simulink model "observerModel_MS"  (R2023b)
settings: Solver=ode15s  StartTime=0.0  StopTime=duration  MaxStep=0.02  RelTol=0.02  AbsTol=0.02  EnableMultiTasking=on
values from neighbouring files (symbols this model uses):
  beta1 = s(8)    [Observer_Optimize.m]
  beta2 = s(7)    [Observer_Optimize.m]
  delta_t = time(2) - time (1)    [Observer_Optimize.m]
  df = 1    [Observer_Optimize.m]
  f_oto = 2    [Observer_Optimize.m]
  f_scc = 2    [Observer_Optimize.m]
  f_visO = 0.2    [Observer_Optimize.m]
  f_visV = 2    [Observer_Optimize.m]
  f_visX = 2    [Observer_Optimize.m]
  GG0 = [0 0 -hypo]'    [Observer_Optimize.m]
  kaa = -2*[1 1 1]'    [Observer_Optimize.m]
  Kea = s(1)^(1/2)*[1 1 1]    [Observer_Optimize.m]
  Kef = s(3)^(1/2)*[1 1 1]    [Observer_Optimize.m]
  Kew = s(2)^(1/2)*[1 1 1]    [Observer_Optimize.m]
  Kfast = s(4)    [Observer_Optimize.m]
  kfg = 1*[1 1 1]'    [Observer_Optimize.m]
  kfw = 1*[1 1 1]'    [Observer_Optimize.m]
  kgvg = 5*[1 1 1]'    [Observer_Optimize.m]
  kwg = 1*[1 1 1]'    [Observer_Optimize.m]
  kwvw = 10*[1 1 1]'    [Observer_Optimize.m]
  kww = 3*[1 1 1]'    [Observer_Optimize.m]
  kxdotva = 0.75*[1 1 1]'    [Observer_Optimize.m]
  kxvv = 0.1*[1 1 1]'    [Observer_Optimize.m]
  ms_exp = s(6)    [Observer_Optimize.m]
  oto_a = 60*[1 1 1]'    [Observer_Optimize.m]
  oto_Ka = 1.3*[1 1 1]'    [Observer_Optimize.m]
  Q0 = [cos(E_angle/2) E(1)*sin(E_angle/2) E(2)*sin(E_angle/2) E(3)*sin(E_angle/2)]'    [Observer_Optimize.m]
  tau_a = tau_a_value*[1 1 1]'    [Observer_Optimize.m]
  tau_scc = tau_scc_value*[1 1 1]'    [Observer_Optimize.m]
  x_leak = 0.6    [Observer_Optimize.m]
  y_leak = 0.6    [Observer_Optimize.m]
  z_leak = 10    [Observer_Optimize.m]
(part 1 of 3)
settings Model: Creator=Newman  LastModifiedBy=aaronallred
settings SolverCC: AutoScaleAbsTol=off  AlgebraicLoopSolver=TrustRegion
settings DataIOCC: SaveFormat=Array  SignalLoggingSaveFormat=ModelDataLogs  SaveOutput=off  SaveTime=off  ReturnWorkspaceOutputs=off
settings OptimizationCC: ExpressionDepthLimit=2147483647  InitFltsAndDblsToZero=on  LifeSpan=inf
settings DebuggingCC: SaveWithParameterizedLinksMsg=none  UnderspecifiedInitializationDetection=Classic  MergeDetectMultiDrivingBlocksExec=none  SolverPrmCheckMsg=warning  FcnCallInpInsideContextMsg=warning  UnconnectedInputMsg=warning  UnconnectedOutputMsg=warning  UnconnectedLineMsg=warning  StateNameClashWarn=warning  SFUnexpectedBacktrackingDiag=warning  SFNoUnconditionalDefaultTransitionDiag=warning  SFExecutionAtInitializationDiag=none  ArithmeticOperatorsInVariantConditions=warning
settings HardwareCC: ProdBitPerPointer=32  ProdBitPerSizeT=32  ProdBitPerPtrDiffT=32  ProdLargestAtomicFloat=None  ProdIntDivRoundTo=Undefined  ProdEndianess=Unspecified  ProdWordSize=32  ProdHWDeviceType=32-bit Generic
settings ModelReferenceCC: EnableRefExpFcnMdlSchedulingChecks=on  PropagateSignalLabelsOutOfModel=off
settings SFSimCC: SimUseLocalCustomCode=off  CustomCodeUndefinedFunction=UseInterfaceOnly
settings RTWCC: RTWUseLocalCustomCode=off  DLArmComputeVersion=19.05
settings CodeAppCC: StateflowObjectComments=on
settings GRTTargetCC: TargetFcnLib=ansi_tfl_tmw.mat  TargetLangStandard=C89/C90 (ANSI)  CombineOutputUpdateFcns=off  GRTInterface=on
settings ConfigComp: CovMetricSettings=dw  CovSaveCumulativeToWorkspaceVar=on  CovSaveSingleToWorkspaceVar=on  CovExternalEMLEnable=off

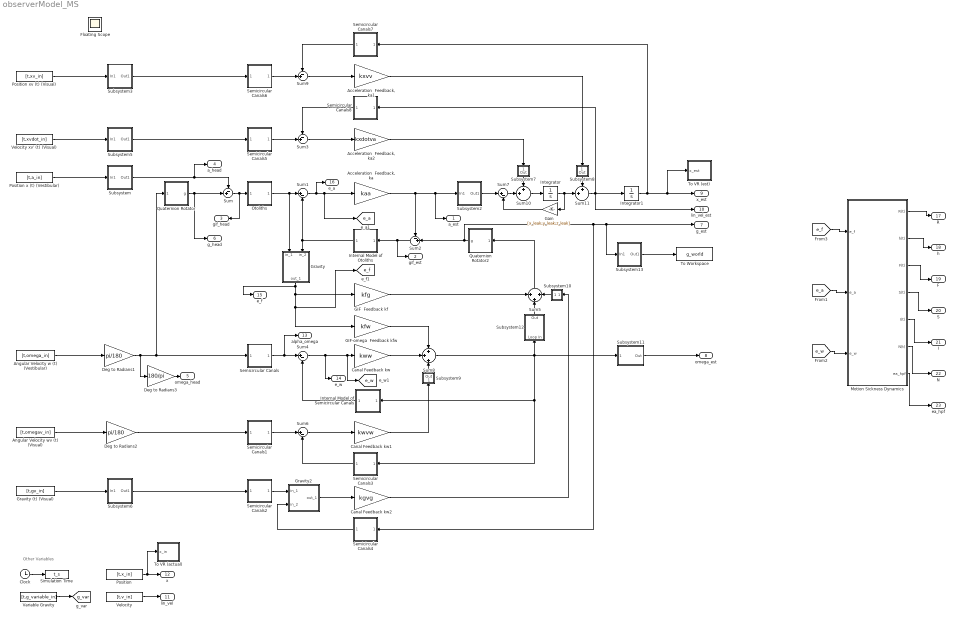
== system observerModel_MS ==
  note: Other Variables
  "Acceleration  Feedback, ka" : Gain  Gain=kaa  SaturateOnIntegerOverflow=on  OutDataTypeStr=Inherit: Same as input  ParamDataTypeStr=Inherit: Same as input
  "Acceleration  Feedback, ka1" : Gain  Gain=kxvv  SaturateOnIntegerOverflow=on  OutDataTypeStr=Inherit: Same as input  ParamDataTypeStr=Inherit: Same as input
  "Acceleration  Feedback, ka2" : Gain  Gain=kxdotva  SaturateOnIntegerOverflow=on  OutDataTypeStr=Inherit: Same as input  ParamDataTypeStr=Inherit: Same as input
  Angular Velocity w (t) (Vestibular) : FromWorkspace  VariableName=[t,omega_in]  ZeroCross=off
  Angular Velocity wv (t) (Visual) : FromWorkspace  VariableName=[t,omegav_in]  ZeroCross=off
  Canal Feedback kw : Gain  Gain=kww  SaturateOnIntegerOverflow=on  OutDataTypeStr=Inherit: Same as input  ParamDataTypeStr=Inherit: Same as input
  Canal Feedback kw1 : Gain  Gain=kwvw  SaturateOnIntegerOverflow=on  OutDataTypeStr=Inherit: Same as input  ParamDataTypeStr=Inherit: Same as input
  Canal Feedback kw2 : Gain  Gain=kgvg  SaturateOnIntegerOverflow=on  OutDataTypeStr=Inherit: Same as input  ParamDataTypeStr=Inherit: Same as input
  Clock : Clock
  Deg to Radians1 : Gain  Gain=pi/180  SaturateOnIntegerOverflow=on  OutDataTypeStr=Inherit: Same as input  ParamDataTypeStr=Inherit: Same as input
  Deg to Radians2 : Gain  Gain=pi/180  SaturateOnIntegerOverflow=on  OutDataTypeStr=Inherit: Same as input  ParamDataTypeStr=Inherit: Same as input
  Deg to Radians3 : Gain  Gain=180/pi  SaturateOnIntegerOverflow=on  OutDataTypeStr=Inherit: Same as input  ParamDataTypeStr=Inherit: Same as input
  GIF  Feedback kf : Gain  Gain=kfg  SaturateOnIntegerOverflow=on  OutDataTypeStr=Inherit: Same as input  ParamDataTypeStr=Inherit: Same as input
  GIF-omega  Feedback kfw : Gain  Gain=kfw  SaturateOnIntegerOverflow=on  OutDataTypeStr=Inherit: Same as input  ParamDataTypeStr=Inherit: Same as input
  Gain : Gain  Gain=[x_leak;y_leak;z_leak]
  Gravity : Subsystem
  Gravity (t) (Visual) : FromWorkspace  VariableName=[t,gv_in]  ZeroCross=off
  Gravity2 : Subsystem
  Integrator : Integrator  InitialCondition=[0;0;-4.432]
  Integrator1 : Integrator  InitialCondition=[0;0;0]
  Internal Model of Otoliths : Subsystem
      mask Display: fprintf('<OTO>')
  Internal Model of Semicircular Canals : Subsystem
      mask Display: fprintf('<SCC>')
  Motion Sickness Dynamics : Subsystem
  Otoliths : Subsystem
      mask Display: fprintf('OTO')
  Position : FromWorkspace  VariableName=[t,x_in]  ZeroCross=off
  Position x (t) (Vestibular) : FromWorkspace  VariableName=[t,a_in]  ZeroCross=off
  Position xv (t) (Visual) : FromWorkspace  VariableName=[t,xv_in]  ZeroCross=off
  Quaternion Rotator : Subsystem
      mask Display: fprintf('G(w)')
  Quaternion Rotator2 : Subsystem
      mask Display: fprintf('Gest(w)')
  Semicircular Canals : Subsystem
      mask Display: fprintf('SCC')
  Semicircular Canals1 : Subsystem
      mask Display: fprintf('VISw')
  Semicircular Canals2 : Subsystem
      mask Display: fprintf('VISg')
  Semicircular Canals3 : Subsystem
      mask Display: fprintf('<VISw>')
  Semicircular Canals4 : Subsystem
      mask Display: fprintf('<VISg>')
  Semicircular Canals5 : Subsystem
      mask Display: fprintf('VISxdot')
  Semicircular Canals6 : Subsystem
      mask Display: fprintf('VISx')
  Semicircular Canals7 : Subsystem
      mask Display: fprintf('<VISx>')
  Semicircular Canals8 : Subsystem
      mask Display: fprintf('<VISxdot>')
  Simulation Time : ToWorkspace  VariableName=t_s
      settings: MaxDataPoints=100000
  Subsystem : Subsystem
      mask Display: fprintf('TH(w)')
  Subsystem10 : Subsystem
      mask Display: fprintf('/')
  Subsystem11 : Subsystem
      mask Display: fprintf('K')
  Subsystem12 : Subsystem
      mask Display: fprintf('K')
  Subsystem13 : Subsystem
      mask Display: fprintf('TW(w_est)')
  Subsystem2 : Subsystem
      mask Display: fprintf('TW(w_est)')
  Subsystem3 : Subsystem
      mask Display: fprintf('T')
  Subsystem5 : Subsystem
      mask Display: fprintf('T')
  Subsystem6 : Subsystem
      mask Display: fprintf('TH(w)')
  Subsystem7 : Subsystem
      mask Display: fprintf('/')
  Subsystem8 : Subsystem
      mask Display: fprintf('/')
  Subsystem9 : Subsystem
      mask Display: fprintf('/')
  Sum{,2..3,9} (4 alike) : Sum  Inputs=-+|
  Sum{1,4,6..7} (4 alike) : Sum  Inputs=|+-
  Sum10 : Sum  Inputs=++|
  Sum11 : Sum  Inputs=++|
  Sum5 : Sum  Inputs=+|+|+
  Sum8 : Sum  Inputs=+|+|+
  To VR (actual) : Subsystem
  To VR (est) : Subsystem
  To Workspace : ToWorkspace  VariableName=g_world  SampleTime=-1
  Variable Gravity : FromWorkspace  VariableName=[t,g_variable_in]  ZeroCross=off
  Velocity : FromWorkspace  VariableName=[t,v_in]  ZeroCross=off
  Velocity xv' (t) (Visual) : FromWorkspace  VariableName=[t,xvdot_in]  ZeroCross=off
  a_est : Outport
  gif_est : Outport  Port=2
  gif_head : Outport  Port=3
  a_head : Outport  Port=4
  omega_head : Outport  Port=5
  g_head : Outport  Port=6
  g_est : Outport  Port=7
  omega_est : Outport  Port=8
  x_est : Outport  Port=9
  lin_vel_est : Outport  Port=10
  lin_vel : Outport  Port=11
  x : Outport  Port=12
  alpha_omega : Outport  Port=13
  e_w : Outport  Port=14
  e_f : Outport  Port=15
  e_a : Outport  Port=16
  R : Outport  Port=17  VectorParamsAs1DForOutWhenUnconnected=off
  h : Outport  Port=18  VectorParamsAs1DForOutWhenUnconnected=off
  F : Outport  Port=19  VectorParamsAs1DForOutWhenUnconnected=off
  S : Outport  Port=20  VectorParamsAs1DForOutWhenUnconnected=off
  I : Outport  Port=21  VectorParamsAs1DForOutWhenUnconnected=off
  N : Outport  Port=22  VectorParamsAs1DForOutWhenUnconnected=off
  ea_hpf : Outport  Port=23
  Floating Scope : Scope
  tag scope: e_a=global, e_f=global, e_w=global, g_var=global
  wires:
  Clock/1 -> Simulation Time/1
  Quaternion Rotator/1(g) -> Sum/2, g_head/1
  Position x (t) (Vestibular)/1 -> Subsystem/1(In1)
  Sum/1 -> gif_head/1, Otoliths/1(Inport)
  Sum1/1 -> [e_a], "Acceleration  Feedback, ka"/1, e_a/1
  Otoliths/1(Outport) -> Sum1/1, Gravity/1(in_1)
  Sum2/1 -> gif_est/1, Internal Model of Otoliths/1(Inport)
  "Acceleration  Feedback, ka"/1 -> Sum2/1, a_est/1, Subsystem2/1(In1)
  Gravity/1(out_1) -> GIF-omega  Feedback kfw/1, [e_f], GIF  Feedback kf/1, e_f/1
  GIF  Feedback kf/1 -> Sum5/1
  Sum5/1 -> Quaternion Rotator2/1(omega_rad_est)
  Sum4/1 -> [e_w], Canal Feedback kw/1, e_w/1
  GIF-omega  Feedback kfw/1 -> Sum8/1
  Canal Feedback kw/1 -> Sum8/2
  Internal Model of Semicircular Canals/1(Outport) -> Sum4/2
  Internal Model of Otoliths/1(Outport) -> Gravity/2(in_2), Sum1/2
  Sum8/1 -> Semicircular Canals3/1(Inport), Internal Model of Semicircular Canals/1(Inport), Subsystem11/1(Loop In), Subsystem12/1(Loop In)
  Quaternion Rotator2/1(g) -> Semicircular Canals4/1(Inport), g_est/1, Subsystem13/1(In1), Sum2/2
  Semicircular Canals/1(Outport) -> alpha_omega/1, Sum4/1
  Angular Velocity w (t) (Vestibular)/1 -> Deg to Radians1/1
  Semicircular Canals1/1(Outport) -> Sum6/1
  Semicircular Canals3/1(Outport) -> Sum6/2
  Sum6/1 -> Canal Feedback kw1/1
  Canal Feedback kw1/1 -> Subsystem9/1(Loop In)
  Semicircular Canals5/1(Outport) -> Sum3/2
  Semicircular Canals6/1(Outport) -> Sum9/2
  Semicircular Canals7/1(Outport) -> Sum9/1
  Semicircular Canals8/1(Outport) -> Sum3/1
  Sum3/1 -> "Acceleration  Feedback, ka2"/1
  Sum9/1 -> "Acceleration  Feedback, ka1"/1
  Sum10/1 -> Integrator/1
  Integrator/1 -> Gain/1, Sum11/2
  Sum11/1 -> Semicircular Canals8/1(Inport), lin_vel_est/1, Integrator1/1
  Integrator1/1 -> Semicircular Canals7/1(Inport), x_est/1, To VR (est)/1(x_est)
  Gravity2/1(out_1) -> Canal Feedback kw2/1
  Velocity xv' (t) (Visual)/1 -> Subsystem5/1(In1)
  Position xv (t) (Visual)/1 -> Subsystem3/1(In1)
  Angular Velocity wv (t) (Visual)/1 -> Deg to Radians2/1
  Deg to Radians2/1 -> Semicircular Canals1/1(Inport)
  Gravity (t) (Visual)/1 -> Subsystem6/1(In1)
  Deg to Radians3/1 -> omega_head/1
  Canal Feedback kw2/1 -> Subsystem10/1(Loop In)
  Subsystem5/1(Out1) -> Semicircular Canals5/1(Inport)
  Subsystem3/1(Out1) -> Semicircular Canals6/1(Inport)
  "Acceleration  Feedback, ka2"/1 -> Subsystem7/1(Loop In)
  "Acceleration  Feedback, ka1"/1 -> Subsystem8/1(Loop In)
  Subsystem7/1(Out) -> Sum10/1
  Subsystem8/1(Out) -> Sum11/1
  Subsystem9/1(Out) -> Sum8/3
  Subsystem10/1(Out) -> Sum5/3
  Sum7/1 -> Sum10/2
  Subsystem2/1(Out1) -> Sum7/1
  Gain/1 -> Sum7/2
  Semicircular Canals4/1(Outport) -> Gravity2/2(in_2)
  Semicircular Canals2/1(Outport) -> Gravity2/1(in_1)
  Variable Gravity/1 -> [g_var]
  Deg to Radians1/1 -> Quaternion Rotator/1(omega_rad), Semicircular Canals/1(Inport), Deg to Radians3/1
  Velocity/1 -> lin_vel/1
  Position/1 -> x/1, To VR (actual)/1(x_in)
  Subsystem6/1(Out1) -> Semicircular Canals2/1(Inport)
  Subsystem/1(Out1) -> Sum/1, a_head/1
  Subsystem13/1(Out1) -> To Workspace/1
  Subsystem11/1(Out) -> omega_est/1
  Subsystem12/1(Out) -> Sum5/2
  [e_w] -> Motion Sickness Dynamics/3(e_w)
  [e_f] -> Motion Sickness Dynamics/1(e_f)
  Motion Sickness Dynamics/3(F(t)) -> F/1
  Motion Sickness Dynamics/5(I(t)) -> I/1
  Motion Sickness Dynamics/2(h(t)) -> h/1
  [e_a] -> Motion Sickness Dynamics/2(e_a)
  Motion Sickness Dynamics/6(N(t)) -> N/1
  Motion Sickness Dynamics/4(S(t)) -> S/1
  Motion Sickness Dynamics/1(R(t)) -> R/1
  Motion Sickness Dynamics/7(ea_hpf) -> ea_hpf/1

== system observerModel_MS/Gravity ==
  in_1 : Inport
  in_2 : Inport  Port=2
  Cross Product : Subsystem  mask(Nick's Library){}
      mask help: Cross Product
      mask Help: Cross Product
      mask Display: disp('--> -->\nu x v')
  Dot Product : DotProduct  OutDataTypeStr=Inherit: Inherit via internal rule
  Normalize : Subsystem
      mask Display: disp('->\nu\n__\n->\n|u|')
  Normalize1 : Subsystem
      mask Display: disp('->\nu\n__\n->\n|u|')
  Normalize2 : Subsystem
      mask Display: disp('->\nu\n__\n->\n|u|')
  Product : Product  InputSameDT=on  RndMeth=Zero  SaturateOnIntegerOverflow=on  OutDataTypeStr=Inherit: Same as first input
  Trigonometric Function : Trigonometry  Operator=acos
  out_1 : Outport  InitialOutput=0
  wires:
  Trigonometric Function/1 -> Product/2
  Product/1 -> out_1/1
  Normalize1/1(out_1) -> Dot Product/1
  Normalize/1(out_1) -> Dot Product/2
  in_1/1 -> Normalize1/1(in_1), Cross Product/1(in_1)
  Normalize2/1(out_1) -> Product/1
  Dot Product/1 -> Trigonometric Function/1
  Cross Product/1(out_1) -> Normalize2/1(in_1)
  in_2/1 -> Normalize/1(in_1), Cross Product/2(in_2)

== system observerModel_MS/Gravity2 ==
  in_1 : Inport
  in_2 : Inport  Port=2
  Cross Product : Subsystem  mask(Nick's Library){}
      mask help: Cross Product
      mask Help: Cross Product
      mask Display: disp('--> -->\nu x v')
  Dot Product : DotProduct  OutDataTypeStr=Inherit: Inherit via internal rule
  Normalize : Subsystem
      mask Display: disp('->\nu\n__\n->\n|u|')
  Normalize1 : Subsystem
      mask Display: disp('->\nu\n__\n->\n|u|')
  Normalize2 : Subsystem
      mask Display: disp('->\nu\n__\n->\n|u|')
  Product : Product  InputSameDT=on  RndMeth=Zero  SaturateOnIntegerOverflow=on  OutDataTypeStr=Inherit: Same as first input
  Trigonometric Function : Trigonometry  Operator=acos
  out_1 : Outport  InitialOutput=0
  wires:
  Trigonometric Function/1 -> Product/2
  Product/1 -> out_1/1
  Normalize1/1(out_1) -> Dot Product/1
  Normalize/1(out_1) -> Dot Product/2
  in_1/1 -> Normalize1/1(in_1), Cross Product/1(in_1)
  Normalize2/1(out_1) -> Product/1
  Dot Product/1 -> Trigonometric Function/1
  Cross Product/1(out_1) -> Normalize2/1(in_1)
  in_2/1 -> Normalize/1(in_1), Cross Product/2(in_2)

== system observerModel_MS/Internal Model of Otoliths ==
  note: Z otolith
  note: Y otolith
  note: X otolith
  Inport : Inport
  Demux : Demux  Outputs=3
      settings: DisplayOption=none
  Mux : Mux  Inputs=3
  Otolith : Subsystem
  Otolith1 : Subsystem
  Otolith2 : Subsystem
  Outport : Outport  InitialOutput=0
  wires:
  Otolith2/1(out_1) -> Mux/3
  Otolith/1(out_1) -> Mux/1
  Otolith1/1(out_1) -> Mux/2
  Demux/3 -> Otolith2/1(in_1)
  Demux/1 -> Otolith/1(in_1)
  Demux/2 -> Otolith1/1(in_1)
  Inport/1 -> Demux/1
  Mux/1 -> Outport/1

== system observerModel_MS/Internal Model of Semicircular Canals ==
  note: Z canal
  note: Y canal
  note: X canal
  Inport : Inport
  Demux : Demux  Outputs=3
      settings: DisplayOption=none
  Mux : Mux  Inputs=3
  Zero-Pole : ZeroPole  Zeros=[0]  Poles=[-1/tau_scc(1);-2*pi*f_scc]  Gain=[(2*pi*f_scc)]
  Zero-Pole1 : ZeroPole  Zeros=[0]  Poles=[-1/tau_scc(2);-2*pi*f_scc]  Gain=[(2*pi*f_scc)]
  Zero-Pole2 : ZeroPole  Zeros=[0]  Poles=[-1/tau_scc(3);-2*pi*f_scc]  Gain=[(2*pi*f_scc)]
  Outport : Outport  InitialOutput=0
  wires:
  Inport/1 -> Demux/1
  Demux/3 -> Zero-Pole2/1
  Demux/1 -> Zero-Pole/1
  Demux/2 -> Zero-Pole1/1
  Zero-Pole2/1 -> Mux/3
  Zero-Pole1/1 -> Mux/2
  Zero-Pole/1 -> Mux/1
  Mux/1 -> Outport/1

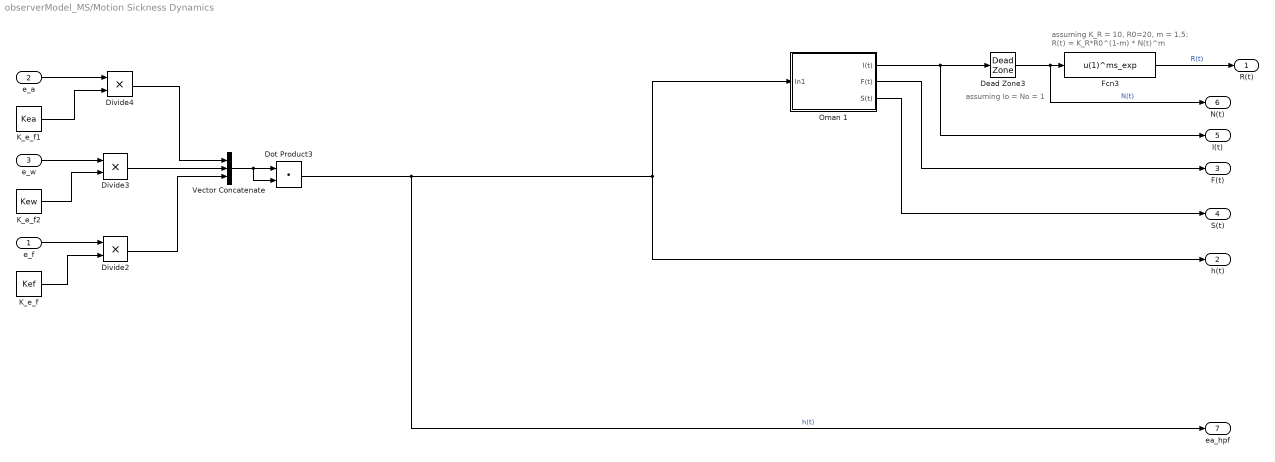
== system observerModel_MS/Motion Sickness Dynamics ==
  note: assuming Io = No = 1
  note: assuming K_R = 10, R0=20, m = 1.5:
      | R(t) = K_R*R0^(1-m) * N(t)^m
  e_f : Inport
  e_a : Inport  Port=2
  e_w : Inport  Port=3
  Dead Zone3 : DeadZone  LowerValue=-100000  UpperValue=dz_end
  Divide2 : Product  Inputs=**
  Divide3 : Product  Inputs=**
  Divide4 : Product  Inputs=**
  Dot Product3 : DotProduct  OutDataTypeStr=Inherit: Inherit via internal rule
  Fcn3 : Fcn  Expr=u(1)^ms_exp
  K_e_f : Constant  Value=Kef
  K_e_f1 : Constant  Value=Kea
  K_e_f2 : Constant  Value=Kew
  Oman 1 : Subsystem
  Vector Concatenate : Concatenate  NumInputs=3
  R(t) : Outport  VectorParamsAs1DForOutWhenUnconnected=off
  h(t) : Outport  Port=2  VectorParamsAs1DForOutWhenUnconnected=off
  F(t) : Outport  Port=3  VectorParamsAs1DForOutWhenUnconnected=off
  S(t) : Outport  Port=4  VectorParamsAs1DForOutWhenUnconnected=off
  I(t) : Outport  Port=5  VectorParamsAs1DForOutWhenUnconnected=off
  N(t) : Outport  Port=6  VectorParamsAs1DForOutWhenUnconnected=off
  ea_hpf : Outport  Port=7
  wires:
  Dot Product3/1 -> h(t)/1, Oman 1/1(In1), ea_hpf/1  "h(t)"
  Dead Zone3/1 -> N(t)/1, Fcn3/1  "N(t)"
  Oman 1/1(I(t)) -> I(t)/1, Dead Zone3/1
  Oman 1/2(F(t)) -> F(t)/1
  Oman 1/3(S(t)) -> S(t)/1
  e_a/1 -> Divide4/1
  Fcn3/1 -> R(t)/1  "R(t)"
  K_e_f/1 -> Divide2/2
  K_e_f1/1 -> Divide4/2
  K_e_f2/1 -> Divide3/2
  e_f/1 -> Divide2/1
  e_w/1 -> Divide3/1
  Divide3/1 -> Vector Concatenate/2
  Divide4/1 -> Vector Concatenate/1
  Divide2/1 -> Vector Concatenate/3
  Vector Concatenate/1 -> Dot Product3/2, Dot Product3/1

== system observerModel_MS/Otoliths ==
  Inport : Inport
  Demux : Demux  Outputs=3
      settings: DisplayOption=none
  Mux : Mux  Inputs=3
  X Graviceptor : Subsystem
  Y Graviceptor : Subsystem
  Z Graviceptor : Subsystem
  Outport : Outport  InitialOutput=0
  wires:
  Z Graviceptor/1(out_1) -> Mux/3
  X Graviceptor/1(out_1) -> Mux/1
  Y Graviceptor/1(out_1) -> Mux/2
  Demux/3 -> Z Graviceptor/1(in_1)
  Demux/1 -> X Graviceptor/1(in_1)
  Demux/2 -> Y Graviceptor/1(in_1)
  Inport/1 -> Demux/1
  Mux/1 -> Outport/1

== system observerModel_MS/Quaternion Rotator ==
  omega_rad : Inport
  Head to Limbic Angular Velocity Transform : Subsystem
  Quaternion Integrator : Subsystem
  Quaternion to Direction Cosine : Subsystem
  Quaternion to Euler Angles : Subsystem
  Rotation : Subsystem
  SVV : ToWorkspace  VariableName=SVV  SampleTime=-1
  Tilt : ToWorkspace  VariableName=tilt  SampleTime=-1
  Tilt & SVV : Subsystem
  To Workspace : ToWorkspace  VariableName=azimuth_head  SampleTime=-1
  To Workspace2 : ToWorkspace  VariableName=euler_head  SampleTime=-1
  g : Outport
  tag scope: D_Cos=global, R_head=global
  wires:
  Quaternion Integrator/1(q) -> Quaternion to Direction Cosine/1(q), Quaternion to Euler Angles/1(q)
  Quaternion to Direction Cosine/1(D_Cos) -> Rotation/1(D_Cos), Head to Limbic Angular Velocity Transform/2(D_Cos), [D_Cos]
  omega_rad/1 -> Quaternion Integrator/1(omega_head), Rotation/2(omega_rad), Head to Limbic Angular Velocity Transform/1(omega_head)
  Rotation/1(g) -> g/1, Tilt & SVV/1(g)
  Rotation/2(azimuth) -> To Workspace/1
  Head to Limbic Angular Velocity Transform/1(R_limbic) -> [R_head]
  Quaternion to Euler Angles/1(Euler) -> To Workspace2/1
  Tilt & SVV/1(Tilt) -> Tilt/1
  Tilt & SVV/2(SVV) -> SVV/1

== system observerModel_MS/Quaternion Rotator2 ==
  omega_rad_est : Inport
  Head to Limbic Angular Velocity Transform Rotation Matrix : Subsystem
  Quaternion Integrator : Subsystem
  Quaternion to Direction Cosine : Subsystem
  Quaternion to Euler Angles : Subsystem
  Rotation : Subsystem
  SVV Est : ToWorkspace  VariableName=SVV_est  SampleTime=-1
  Tilt & SVV : Subsystem
  Tilt Est : ToWorkspace  VariableName=tilt_est  SampleTime=-1
  To Workspace : ToWorkspace  VariableName=azimuth_est  SampleTime=-1
  To Workspace2 : ToWorkspace  VariableName=euler_est  SampleTime=-1
  g : Outport
  tag scope: D_Cos_est=global, R_est=global
  wires:
  Quaternion Integrator/1(q) -> Quaternion to Direction Cosine/1(q), Quaternion to Euler Angles/1(q)
  Quaternion to Direction Cosine/1(D_Cos) -> Rotation/1(D_Cos), [D_Cos_est], Head to Limbic Angular Velocity Transform Rotation Matrix/2(D_Cos)
  omega_rad_est/1 -> Quaternion Integrator/1(omega_rad_est), Rotation/2(omega_rad), Head to Limbic Angular Velocity Transform Rotation Matrix/1(omega_est)
  Rotation/1(g) -> g/1, Tilt & SVV/1(g)
  Rotation/2(azimuth) -> To Workspace/1
  Head to Limbic Angular Velocity Transform Rotation Matrix/1(R_limbic_est) -> [R_est]
  Quaternion to Euler Angles/1(Euler) -> To Workspace2/1
  Tilt & SVV/1(Tilt) -> Tilt Est/1
  Tilt & SVV/2(SVV) -> SVV Est/1

== system observerModel_MS/Semicircular Canals ==
  note: Z canal
  note: Y canal
  note: X canal
  Inport : Inport
  Demux : Demux  Outputs=3
      settings: DisplayOption=none
  Mux : Mux  Inputs=3
  Zero-Pole : ZeroPole  Zeros=[0;0]  Poles=[-1/tau_scc(1);-1/tau_a(1);-2*pi*f_scc]  Gain=[(2*pi*f_scc)]
  Zero-Pole1 : ZeroPole  Zeros=[0;0]  Poles=[-1/tau_scc(2);-1/tau_a(2);-2*pi*f_scc]  Gain=[(2*pi*f_scc)]
  Zero-Pole2 : ZeroPole  Zeros=[0;0]  Poles=[-1/tau_scc(3);-1/tau_a(3);-2*pi*f_scc]  Gain=[(2*pi*f_scc)]
  Outport : Outport  InitialOutput=0
  wires:
  Demux/3 -> Zero-Pole2/1
  Demux/1 -> Zero-Pole/1
  Demux/2 -> Zero-Pole1/1
  Zero-Pole2/1 -> Mux/3
  Zero-Pole1/1 -> Mux/2
  Zero-Pole/1 -> Mux/1
  Inport/1 -> Demux/1
  Mux/1 -> Outport/1

== system observerModel_MS/Semicircular Canals1 ==
  Inport : Inport
  Deg to Radians4 : Gain  Gain=-1  SaturateOnIntegerOverflow=on  OutDataTypeStr=Inherit: Same as input  ParamDataTypeStr=Inherit: Same as input
  Demux : Demux  Outputs=3
      settings: DisplayOption=none
  Low Pass Filter : TransferFcn  Denominator=[1/(2*pi*f_visO) 1]
  Low Pass Filter1 : TransferFcn  Denominator=[1/(2*pi*f_visO) 1]
  Low Pass Filter2 : TransferFcn  Denominator=[1/(2*pi*f_visO) 1]
  Mux : Mux  Inputs=3
  Outport : Outport  InitialOutput=0
  wires:
  Inport/1 -> Deg to Radians4/1
  Mux/1 -> Outport/1
  Demux/1 -> Low Pass Filter/1
  Low Pass Filter/1 -> Mux/1
  Demux/3 -> Low Pass Filter2/1
  Demux/2 -> Low Pass Filter1/1
  Low Pass Filter1/1 -> Mux/2
  Low Pass Filter2/1 -> Mux/3
  Deg to Radians4/1 -> Demux/1

== system observerModel_MS/Semicircular Canals2 ==
  Inport : Inport
  Outport : Outport  InitialOutput=0
  wires:
  Inport/1 -> Outport/1

== system observerModel_MS/Semicircular Canals3 ==
  Inport : Inport
  Demux : Demux  Outputs=3
      settings: DisplayOption=none
  Low Pass Filter : TransferFcn  Denominator=[1/(2*pi*f_visO) 1]
  Low Pass Filter1 : TransferFcn  Denominator=[1/(2*pi*f_visO) 1]
  Low Pass Filter2 : TransferFcn  Denominator=[1/(2*pi*f_visO) 1]
  Mux : Mux  Inputs=3
  Outport : Outport  InitialOutput=0
  wires:
  Inport/1 -> Demux/1
  Mux/1 -> Outport/1
  Demux/1 -> Low Pass Filter/1
  Low Pass Filter/1 -> Mux/1
  Demux/3 -> Low Pass Filter2/1
  Demux/2 -> Low Pass Filter1/1
  Low Pass Filter1/1 -> Mux/2
  Low Pass Filter2/1 -> Mux/3

== system observerModel_MS/Semicircular Canals4 ==
  Inport : Inport
  Outport : Outport  InitialOutput=0
  wires:
  Inport/1 -> Outport/1

== system observerModel_MS/Semicircular Canals5 ==
  Inport : Inport
  Deg to Radians4 : Gain  Gain=-1  SaturateOnIntegerOverflow=on  OutDataTypeStr=Inherit: Same as input  ParamDataTypeStr=Inherit: Same as input
  Demux : Demux  Outputs=3
      settings: DisplayOption=none
  Low Pass Filter : TransferFcn  Denominator=[1/(2*pi*f_visV) 1]
  Low Pass Filter1 : TransferFcn  Denominator=[1/(2*pi*f_visV) 1]
  Low Pass Filter2 : TransferFcn  Denominator=[1/(2*pi*f_visV) 1]
  Mux : Mux  Inputs=3
  Outport : Outport  InitialOutput=0
  wires:
  Inport/1 -> Deg to Radians4/1
  Mux/1 -> Outport/1
  Demux/1 -> Low Pass Filter/1
  Low Pass Filter/1 -> Mux/1
  Demux/3 -> Low Pass Filter2/1
  Demux/2 -> Low Pass Filter1/1
  Low Pass Filter1/1 -> Mux/2
  Low Pass Filter2/1 -> Mux/3
  Deg to Radians4/1 -> Demux/1

== system observerModel_MS/Semicircular Canals6 ==
  Inport : Inport
  Demux : Demux  Outputs=3
      settings: DisplayOption=none
  Low Pass Filter : TransferFcn  Denominator=[1/(2*pi*f_visX) 1]
  Low Pass Filter1 : TransferFcn  Denominator=[1/(2*pi*f_visX) 1]
  Low Pass Filter2 : TransferFcn  Denominator=[1/(2*pi*f_visX) 1]
  Mux : Mux  Inputs=3
  Outport : Outport  InitialOutput=0
  wires:
  Inport/1 -> Demux/1
  Mux/1 -> Outport/1
  Demux/1 -> Low Pass Filter/1
  Low Pass Filter/1 -> Mux/1
  Demux/3 -> Low Pass Filter2/1
  Demux/2 -> Low Pass Filter1/1
  Low Pass Filter1/1 -> Mux/2
  Low Pass Filter2/1 -> Mux/3

== system observerModel_MS/Semicircular Canals7 ==
  Inport : Inport
  Demux : Demux  Outputs=3
      settings: DisplayOption=none
  Low Pass Filter : TransferFcn  Denominator=[1/(2*pi*f_visX) 1]
  Low Pass Filter1 : TransferFcn  Denominator=[1/(2*pi*f_visX) 1]
  Low Pass Filter2 : TransferFcn  Denominator=[1/(2*pi*f_visX) 1]
  Mux : Mux  Inputs=3
  Outport : Outport  InitialOutput=0
  wires:
  Inport/1 -> Demux/1
  Mux/1 -> Outport/1
  Demux/1 -> Low Pass Filter/1
  Low Pass Filter/1 -> Mux/1
  Demux/3 -> Low Pass Filter2/1
  Demux/2 -> Low Pass Filter1/1
  Low Pass Filter1/1 -> Mux/2
  Low Pass Filter2/1 -> Mux/3

== system observerModel_MS/Semicircular Canals8 ==
  Inport : Inport
  Demux : Demux  Outputs=3
      settings: DisplayOption=none
  Low Pass Filter : TransferFcn  Denominator=[1/(2*pi*f_visV) 1]
  Low Pass Filter1 : TransferFcn  Denominator=[1/(2*pi*f_visV) 1]
  Low Pass Filter2 : TransferFcn  Denominator=[1/(2*pi*f_visV) 1]
  Mux : Mux  Inputs=3
  Outport : Outport  InitialOutput=0
  wires:
  Inport/1 -> Demux/1
  Mux/1 -> Outport/1
  Demux/1 -> Low Pass Filter/1
  Low Pass Filter/1 -> Mux/1
  Demux/3 -> Low Pass Filter2/1
  Demux/2 -> Low Pass Filter1/1
  Low Pass Filter1/1 -> Mux/2
  Low Pass Filter2/1 -> Mux/3

== system observerModel_MS/Subsystem ==
  In1 : Inport
  Deg to Radians4 : Gain  Gain=1/9.80665  SaturateOnIntegerOverflow=on  OutDataTypeStr=Inherit: Same as input  ParamDataTypeStr=Inherit: Same as input
  Matrix Multiplication : Subsystem
  Out1 : Outport
  wires:
  [D_Cos] -> Matrix Multiplication/1(D_Cos)
  In1/1 -> Deg to Radians4/1
  Matrix Multiplication/1(a_head) -> Out1/1
  Deg to Radians4/1 -> Matrix Multiplication/2(a_world)

== system observerModel_MS/Subsystem10 ==
  Loop In : Inport
  Gravity Switch : FromWorkspace  VariableName=[t,g_ON]  ZeroCross=off
  If Input Equals Kill Signal Value Evaluate a 1 : RelationalOperator  Operator===  OutDataTypeStr=boolean  InputSameDT=off
  If This Recieves a 1 Pass Top Signal : Switch  Criteria=u2 ~= 0  SaturateOnIntegerOverflow=off  InputSameDT=off
  Kill Signal Value : Constant  Value=0
  Signal = 0 : Constant  Value=0
  To Workspace : ToWorkspace  VariableName=gv_switch  SampleTime=-1
  Out : Outport
  wires:
  If Input Equals Kill Signal Value Evaluate a 1/1 -> If This Recieves a 1 Pass Top Signal/2, To Workspace/1
  Signal = 0/1 -> If This Recieves a 1 Pass Top Signal/1
  If This Recieves a 1 Pass Top Signal/1 -> Out/1
  Kill Signal Value/1 -> If Input Equals Kill Signal Value Evaluate a 1/1
  Loop In/1 -> If This Recieves a 1 Pass Top Signal/3
  Gravity Switch/1 -> If Input Equals Kill Signal Value Evaluate a 1/2

== system observerModel_MS/Subsystem11 ==
  Loop In : Inport
  (Kwf+1)/Kwf : Gain  Gain=((kww+kwvw+1)./(kww+kwvw))  SaturateOnIntegerOverflow=on  OutDataTypeStr=Inherit: Same as input  ParamDataTypeStr=Inherit: Same as input
  (Kwf+1)/Kwf1 : Gain  Gain=((kww+1)./(kww))  SaturateOnIntegerOverflow=on  OutDataTypeStr=Inherit: Same as input  ParamDataTypeStr=Inherit: Same as input
  Gravity Switch : FromWorkspace  VariableName=[t,angVel_ON]  ZeroCross=off
  If Input Equals Kill Signal Value Evaluate a 1 : RelationalOperator  Operator===  OutDataTypeStr=boolean  InputSameDT=off
  If This Recieves a 1 Pass Top Signal : Switch  Criteria=u2 ~= 0  SaturateOnIntegerOverflow=off  InputSameDT=off
  Kill Signal Value : Constant  Value=0
  Out : Outport
  wires:
  If Input Equals Kill Signal Value Evaluate a 1/1 -> If This Recieves a 1 Pass Top Signal/2
  If This Recieves a 1 Pass Top Signal/1 -> Out/1
  Loop In/1 -> (Kwf+1)/Kwf1/1, (Kwf+1)/Kwf/1
  Kill Signal Value/1 -> If Input Equals Kill Signal Value Evaluate a 1/1
  Gravity Switch/1 -> If Input Equals Kill Signal Value Evaluate a 1/2
  (Kwf+1)/Kwf/1 -> If This Recieves a 1 Pass Top Signal/3
  (Kwf+1)/Kwf1/1 -> If This Recieves a 1 Pass Top Signal/1

== system observerModel_MS/Subsystem12 ==
  Loop In : Inport
  (Kwf+1)/Kwf : Gain  Gain=kwg.*((kww+kwvw+1)./(kww+kwvw))  SaturateOnIntegerOverflow=on  OutDataTypeStr=Inherit: Same as input  ParamDataTypeStr=Inherit: Same as input
  (Kwf+1)/Kwf1 : Gain  Gain=kwg.*((kww+1)./(kww))  SaturateOnIntegerOverflow=on  OutDataTypeStr=Inherit: Same as input  ParamDataTypeStr=Inherit: Same as input
  Gravity Switch : FromWorkspace  VariableName=[t,angVel_ON]  ZeroCross=off
  If Input Equals Kill Signal Value Evaluate a 1 : RelationalOperator  Operator===  OutDataTypeStr=boolean  InputSameDT=off
  If This Recieves a 1 Pass Top Signal : Switch  Criteria=u2 ~= 0  SaturateOnIntegerOverflow=off  InputSameDT=off
  Kill Signal Value : Constant  Value=0
  Out : Outport
  wires:
  If Input Equals Kill Signal Value Evaluate a 1/1 -> If This Recieves a 1 Pass Top Signal/2
  If This Recieves a 1 Pass Top Signal/1 -> Out/1
  Loop In/1 -> (Kwf+1)/Kwf/1, (Kwf+1)/Kwf1/1
  Kill Signal Value/1 -> If Input Equals Kill Signal Value Evaluate a 1/1
  Gravity Switch/1 -> If Input Equals Kill Signal Value Evaluate a 1/2
  (Kwf+1)/Kwf/1 -> If This Recieves a 1 Pass Top Signal/3
  (Kwf+1)/Kwf1/1 -> If This Recieves a 1 Pass Top Signal/1

== system observerModel_MS/Subsystem13 ==
  In1 : Inport
  Matrix Multiplication : Subsystem
  Out1 : Outport
  wires:
  [D_Cos_est] -> Matrix Multiplication/1(D_Cos)
  Matrix Multiplication/1(a_est_world) -> Out1/1
  In1/1 -> Matrix Multiplication/2(a_esr_head)

== system observerModel_MS/Subsystem2 ==
  In1 : Inport
  Deg to Radians4 : Gain  Gain=9.80665  SaturateOnIntegerOverflow=on  OutDataTypeStr=Inherit: Same as input  ParamDataTypeStr=Inherit: Same as input
  Matrix Multiplication : Subsystem
  Out1 : Outport
  wires:
  [D_Cos_est] -> Matrix Multiplication/1(D_Cos)
  Deg to Radians4/1 -> Out1/1
  Matrix Multiplication/1(a_est_world) -> Deg to Radians4/1
  In1/1 -> Matrix Multiplication/2(a_est_head)

== system observerModel_MS/Subsystem3 ==
  In1 : Inport
  Subsystem3 : Subsystem
      mask Display: fprintf('TH(w)')
  Subsystem4 : Subsystem
      mask Display: fprintf('TW(w_est)')
  Out1 : Outport
  tag scope: Switch_xv=global
  wires:
  Subsystem3/1(Out1) -> Subsystem4/1(In1)
  In1/1 -> Subsystem3/1(In1), [Switch_xv]
  Subsystem4/1(Out1) -> Out1/1

== system observerModel_MS/Subsystem5 ==
  In1 : Inport
  Subsystem3 : Subsystem
      mask Display: fprintf('TH(w)')
  Subsystem4 : Subsystem
      mask Display: fprintf('TW(w_est)')
  Out1 : Outport
  tag scope: Switch_xvdot=global
  wires:
  Subsystem3/1(Out1) -> Subsystem4/1(In1)
  In1/1 -> Subsystem3/1(In1), [Switch_xvdot]
  Subsystem4/1(Out1) -> Out1/1

== system observerModel_MS/Subsystem6 ==
  In1 : Inport
  Matrix Multiplication : Subsystem
  Out1 : Outport
  wires:
  [D_Cos] -> Matrix Multiplication/1(D_Cos)
  Matrix Multiplication/1(a_head) -> Out1/1
  In1/1 -> Matrix Multiplication/2(a_world)

== system observerModel_MS/Subsystem7 ==
  Loop In : Inport
  Gravity Switch : FromWorkspace  VariableName=[t,vel_ON]  ZeroCross=off
  If Input Equals Kill Signal Value Evaluate a 1 : RelationalOperator  Operator===  OutDataTypeStr=boolean  InputSameDT=off
  If This Recieves a 1 Pass Top Signal : Switch  Criteria=u2 ~= 0  SaturateOnIntegerOverflow=off  InputSameDT=off
  Kill Signal Value : Constant  Value=0
  Scope : Scope
  Signal = 0 : Constant  Value=0
  To Workspace : ToWorkspace  VariableName=xvdot_switch  SampleTime=-1
  Out : Outport
  wires:
  If Input Equals Kill Signal Value Evaluate a 1/1 -> If This Recieves a 1 Pass Top Signal/2, Scope/1, To Workspace/1
  Signal = 0/1 -> If This Recieves a 1 Pass Top Signal/1
  If This Recieves a 1 Pass Top Signal/1 -> Out/1
  Loop In/1 -> If This Recieves a 1 Pass Top Signal/3
  Kill Signal Value/1 -> If Input Equals Kill Signal Value Evaluate a 1/1
  Gravity Switch/1 -> If Input Equals Kill Signal Value Evaluate a 1/2

== system observerModel_MS/Subsystem8 ==
  Loop In : Inport
  Gravity Switch : FromWorkspace  VariableName=[t,pos_ON]  ZeroCross=off
  If Input Equals Kill Signal Value Evaluate a 1 : RelationalOperator  Operator===  OutDataTypeStr=boolean  InputSameDT=off
  If This Recieves a 1 Pass Top Signal : Switch  Criteria=u2 ~= 0  SaturateOnIntegerOverflow=off  InputSameDT=off
  Kill Signal Value : Constant  Value=0
  Signal = 0 : Constant  Value=0
  To Workspace : ToWorkspace  VariableName=xv_switch  SampleTime=-1
  Out : Outport
  wires:
  If Input Equals Kill Signal Value Evaluate a 1/1 -> If This Recieves a 1 Pass Top Signal/2, To Workspace/1
  Signal = 0/1 -> If This Recieves a 1 Pass Top Signal/1
  If This Recieves a 1 Pass Top Signal/1 -> Out/1
  Loop In/1 -> If This Recieves a 1 Pass Top Signal/3
  Kill Signal Value/1 -> If Input Equals Kill Signal Value Evaluate a 1/1
  Gravity Switch/1 -> If Input Equals Kill Signal Value Evaluate a 1/2

== system observerModel_MS/Subsystem9 ==
  Loop In : Inport
  Gravity Switch : FromWorkspace  VariableName=[t,angVel_ON]  ZeroCross=off
  If Input Equals Kill Signal Value Evaluate a 1 : RelationalOperator  Operator===  OutDataTypeStr=boolean  InputSameDT=off
  If This Recieves a 1 Pass Top Signal : Switch  Criteria=u2 ~= 0  SaturateOnIntegerOverflow=off  InputSameDT=off
  Kill Signal Value : Constant  Value=0
  Signal = 0 : Constant  Value=0
  To Workspace : ToWorkspace  VariableName=omegav_switch  SampleTime=-1
  Out : Outport
  wires:
  If Input Equals Kill Signal Value Evaluate a 1/1 -> If This Recieves a 1 Pass Top Signal/2, To Workspace/1
  Signal = 0/1 -> If This Recieves a 1 Pass Top Signal/1
  If This Recieves a 1 Pass Top Signal/1 -> Out/1
  Loop In/1 -> If This Recieves a 1 Pass Top Signal/3
  Kill Signal Value/1 -> If Input Equals Kill Signal Value Evaluate a 1/1
  Gravity Switch/1 -> If Input Equals Kill Signal Value Evaluate a 1/2

== system observerModel_MS/To VR (actual) ==
  x_in : Inport
  Limbic to VR Displacement : Subsystem
  tag scope: Disp_head=global
  wires:
  Limbic to VR Displacement/1(VR Displacement) -> [Disp_head]
  x_in/1 -> Limbic to VR Displacement/1(Limbic Displacement)

== system observerModel_MS/To VR (est) ==
  x_est : Inport
  Limbic to VR Estimated Displacement : Subsystem
  tag scope: Disp_est=global
  wires:
  Limbic to VR Estimated Displacement/1(VR Est Displacement) -> [Disp_est]
  x_est/1 -> Limbic to VR Estimated Displacement/1(Limbic Est Displacement)

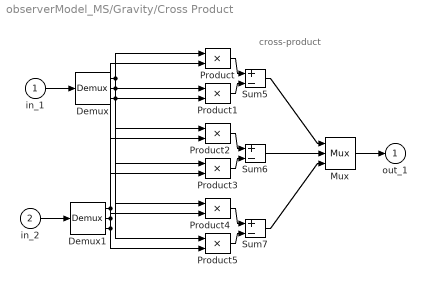
== system observerModel_MS/Gravity/Cross Product ==
  note: cross-product
  in_1 : Inport
  in_2 : Inport  Port=2
  Demux : Demux  Outputs=3
      settings: DisplayOption=none
  Demux1 : Demux  Outputs=3
      settings: DisplayOption=none
  Mux : Mux  Inputs=3
  Product{,1..5} (6 alike) : Product  InputSameDT=on  RndMeth=Zero  SaturateOnIntegerOverflow=on  OutDataTypeStr=Inherit: Same as first input
  Sum5 : Sum  Inputs=+-  InputSameDT=on  SaturateOnIntegerOverflow=on  OutDataTypeStr=Inherit: Same as first input
  Sum6 : Sum  Inputs=+-  InputSameDT=on  SaturateOnIntegerOverflow=on  OutDataTypeStr=Inherit: Same as first input
  Sum7 : Sum  Inputs=+-  InputSameDT=on  SaturateOnIntegerOverflow=on  OutDataTypeStr=Inherit: Same as first input
  out_1 : Outport  InitialOutput=0
  wires:
  in_2/1 -> Demux1/1
  Mux/1 -> out_1/1
  in_1/1 -> Demux/1
  Product/1 -> Sum5/1
  Product1/1 -> Sum5/2
  Product2/1 -> Sum6/1
  Product3/1 -> Sum6/2
  Product4/1 -> Sum7/1
  Product5/1 -> Sum7/2
  Sum5/1 -> Mux/1
  Sum6/1 -> Mux/2
  Sum7/1 -> Mux/3
  Demux/3 -> Product1/1, Product2/1
  Demux1/3 -> Product/2, Product3/2
  Demux/1 -> Product3/1, Product4/1
  Demux1/2 -> Product1/2, Product4/2
  Demux/2 -> Product/1, Product5/1
  Demux1/1 -> Product2/2, Product5/2

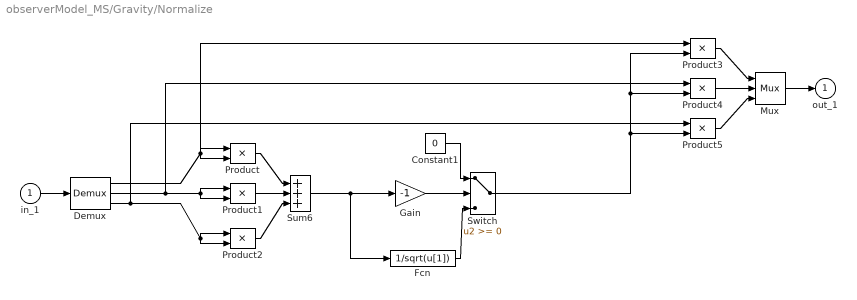
== system observerModel_MS/Gravity/Normalize ==
  in_1 : Inport
  Constant1 : Constant  Value=0
  Demux : Demux  Outputs=3
      settings: DisplayOption=none
  Fcn : Fcn  Expr=1/sqrt(u[1])
  Gain : Gain  Gain=-1  SaturateOnIntegerOverflow=on  OutDataTypeStr=Inherit: Same as input  ParamDataTypeStr=Inherit: Same as input
  Mux : Mux  Inputs=3
  Product{,1..5} (6 alike) : Product  InputSameDT=on  RndMeth=Zero  SaturateOnIntegerOverflow=on  OutDataTypeStr=Inherit: Same as first input
  Sum6 : Sum  Inputs=+++  InputSameDT=on  SaturateOnIntegerOverflow=on  OutDataTypeStr=Inherit: Same as first input
  Switch : Switch
  out_1 : Outport  InitialOutput=0
  wires:
  Sum6/1 -> Gain/1, Fcn/1
  Fcn/1 -> Switch/3
  Constant1/1 -> Switch/1
  Switch/1 -> Product5/2, Product3/2, Product4/2
  Product5/1 -> Mux/3
  Product3/1 -> Mux/1
  Product4/1 -> Mux/2
  Demux/2 -> Product4/1, Product1/1, Product1/2
  Demux/3 -> Product5/1, Product2/2, Product2/1
  Demux/1 -> Product/2, Product/1, Product3/1
  Product1/1 -> Sum6/2
  Product/1 -> Sum6/1
  Product2/1 -> Sum6/3
  Mux/1 -> out_1/1
  in_1/1 -> Demux/1
  Gain/1 -> Switch/2

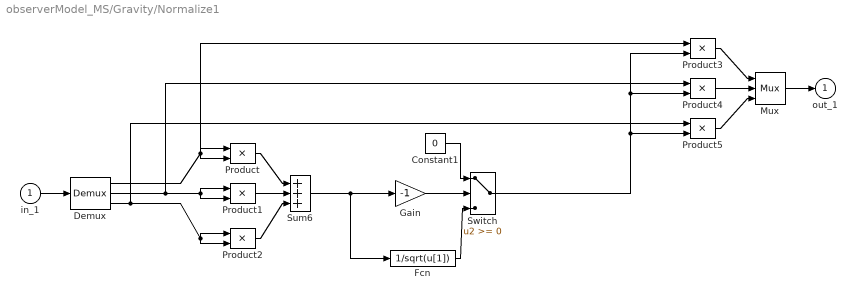
== system observerModel_MS/Gravity/Normalize1 ==
  in_1 : Inport
  Constant1 : Constant  Value=0
  Demux : Demux  Outputs=3
      settings: DisplayOption=none
  Fcn : Fcn  Expr=1/sqrt(u[1])
  Gain : Gain  Gain=-1  SaturateOnIntegerOverflow=on  OutDataTypeStr=Inherit: Same as input  ParamDataTypeStr=Inherit: Same as input
  Mux : Mux  Inputs=3
  Product{,1..5} (6 alike) : Product  InputSameDT=on  RndMeth=Zero  SaturateOnIntegerOverflow=on  OutDataTypeStr=Inherit: Same as first input
  Sum6 : Sum  Inputs=+++  InputSameDT=on  SaturateOnIntegerOverflow=on  OutDataTypeStr=Inherit: Same as first input
  Switch : Switch
  out_1 : Outport  InitialOutput=0
  wires:
  Sum6/1 -> Gain/1, Fcn/1
  Fcn/1 -> Switch/3
  Constant1/1 -> Switch/1
  Switch/1 -> Product5/2, Product3/2, Product4/2
  Product5/1 -> Mux/3
  Product3/1 -> Mux/1
  Product4/1 -> Mux/2
  Demux/2 -> Product4/1, Product1/1, Product1/2
  Demux/3 -> Product5/1, Product2/2, Product2/1
  Demux/1 -> Product/2, Product/1, Product3/1
  Product1/1 -> Sum6/2
  Product/1 -> Sum6/1
  Product2/1 -> Sum6/3
  Mux/1 -> out_1/1
  in_1/1 -> Demux/1
  Gain/1 -> Switch/2

== system observerModel_MS/Gravity/Normalize2 ==
  in_1 : Inport
  Constant1 : Constant  Value=inf
  Demux : Demux  Outputs=3
      settings: DisplayOption=none
  Fcn : Fcn  Expr=1/sqrt(u)
  Gain : Gain  Gain=-1  SaturateOnIntegerOverflow=on  OutDataTypeStr=Inherit: Same as input  ParamDataTypeStr=Inherit: Same as input
  Mux : Mux  Inputs=3
  Product{,1..5} (6 alike) : Product  InputSameDT=on  RndMeth=Zero  SaturateOnIntegerOverflow=on  OutDataTypeStr=Inherit: Same as first input
  Sum6 : Sum  Inputs=+++  InputSameDT=on  SaturateOnIntegerOverflow=on  OutDataTypeStr=Inherit: Same as first input
  Switch : Switch
  out_1 : Outport  InitialOutput=0
  wires:
  Sum6/1 -> Gain/1, Switch/3
  Constant1/1 -> Switch/1
  Product5/1 -> Mux/3
  Product3/1 -> Mux/1
  Product4/1 -> Mux/2
  Demux/2 -> Product4/1, Product1/1, Product1/2
  Demux/3 -> Product5/1, Product2/2, Product2/1
  Demux/1 -> Product/2, Product/1, Product3/1
  Product1/1 -> Sum6/2
  Product/1 -> Sum6/1
  Product2/1 -> Sum6/3
  Mux/1 -> out_1/1
  in_1/1 -> Demux/1
  Gain/1 -> Switch/2
  Switch/1 -> Fcn/1
  Fcn/1 -> Product5/2, Product3/2, Product4/2

== system observerModel_MS/Gravity2/Cross Product ==
  note: cross-product
  in_1 : Inport
  in_2 : Inport  Port=2
  Demux : Demux  Outputs=3
      settings: DisplayOption=none
  Demux1 : Demux  Outputs=3
      settings: DisplayOption=none
  Mux : Mux  Inputs=3
  Product{,1..5} (6 alike) : Product  InputSameDT=on  RndMeth=Zero  SaturateOnIntegerOverflow=on  OutDataTypeStr=Inherit: Same as first input
  Sum5 : Sum  Inputs=+-  InputSameDT=on  SaturateOnIntegerOverflow=on  OutDataTypeStr=Inherit: Same as first input
  Sum6 : Sum  Inputs=+-  InputSameDT=on  SaturateOnIntegerOverflow=on  OutDataTypeStr=Inherit: Same as first input
  Sum7 : Sum  Inputs=+-  InputSameDT=on  SaturateOnIntegerOverflow=on  OutDataTypeStr=Inherit: Same as first input
  out_1 : Outport  InitialOutput=0
  wires:
  in_2/1 -> Demux1/1
  Mux/1 -> out_1/1
  in_1/1 -> Demux/1
  Product/1 -> Sum5/1
  Product1/1 -> Sum5/2
  Product2/1 -> Sum6/1
  Product3/1 -> Sum6/2
  Product4/1 -> Sum7/1
  Product5/1 -> Sum7/2
  Sum5/1 -> Mux/1
  Sum6/1 -> Mux/2
  Sum7/1 -> Mux/3
  Demux/3 -> Product1/1, Product2/1
  Demux1/3 -> Product/2, Product3/2
  Demux/1 -> Product3/1, Product4/1
  Demux1/2 -> Product1/2, Product4/2
  Demux/2 -> Product/1, Product5/1
  Demux1/1 -> Product2/2, Product5/2

== system observerModel_MS/Gravity2/Normalize ==
  in_1 : Inport
  Constant1 : Constant  Value=0
  Demux : Demux  Outputs=3
      settings: DisplayOption=none
  Fcn : Fcn  Expr=1/sqrt(u[1])
  Gain : Gain  Gain=-1  SaturateOnIntegerOverflow=on  OutDataTypeStr=Inherit: Same as input  ParamDataTypeStr=Inherit: Same as input
  Mux : Mux  Inputs=3
  Product{,1..5} (6 alike) : Product  InputSameDT=on  RndMeth=Zero  SaturateOnIntegerOverflow=on  OutDataTypeStr=Inherit: Same as first input
  Sum6 : Sum  Inputs=+++  InputSameDT=on  SaturateOnIntegerOverflow=on  OutDataTypeStr=Inherit: Same as first input
  Switch : Switch
  out_1 : Outport  InitialOutput=0
  wires:
  Sum6/1 -> Gain/1, Fcn/1
  Fcn/1 -> Switch/3
  Constant1/1 -> Switch/1
  Switch/1 -> Product5/2, Product3/2, Product4/2
  Product5/1 -> Mux/3
  Product3/1 -> Mux/1
  Product4/1 -> Mux/2
  Demux/2 -> Product4/1, Product1/1, Product1/2
  Demux/3 -> Product5/1, Product2/2, Product2/1
  Demux/1 -> Product/2, Product/1, Product3/1
  Product1/1 -> Sum6/2
  Product/1 -> Sum6/1
  Product2/1 -> Sum6/3
  Mux/1 -> out_1/1
  in_1/1 -> Demux/1
  Gain/1 -> Switch/2

== system observerModel_MS/Gravity2/Normalize1 ==
  in_1 : Inport
  Constant1 : Constant  Value=0
  Demux : Demux  Outputs=3
      settings: DisplayOption=none
  Fcn : Fcn  Expr=1/sqrt(u[1])
  Gain : Gain  Gain=-1  SaturateOnIntegerOverflow=on  OutDataTypeStr=Inherit: Same as input  ParamDataTypeStr=Inherit: Same as input
  Mux : Mux  Inputs=3
  Product{,1..5} (6 alike) : Product  InputSameDT=on  RndMeth=Zero  SaturateOnIntegerOverflow=on  OutDataTypeStr=Inherit: Same as first input
  Sum6 : Sum  Inputs=+++  InputSameDT=on  SaturateOnIntegerOverflow=on  OutDataTypeStr=Inherit: Same as first input
  Switch : Switch
  out_1 : Outport  InitialOutput=0
  wires:
  Sum6/1 -> Gain/1, Fcn/1
  Fcn/1 -> Switch/3
  Constant1/1 -> Switch/1
  Switch/1 -> Product5/2, Product3/2, Product4/2
  Product5/1 -> Mux/3
  Product3/1 -> Mux/1
  Product4/1 -> Mux/2
  Demux/2 -> Product4/1, Product1/1, Product1/2
  Demux/3 -> Product5/1, Product2/2, Product2/1
  Demux/1 -> Product/2, Product/1, Product3/1
  Product1/1 -> Sum6/2
  Product/1 -> Sum6/1
  Product2/1 -> Sum6/3
  Mux/1 -> out_1/1
  in_1/1 -> Demux/1
  Gain/1 -> Switch/2

== system observerModel_MS/Gravity2/Normalize2 ==
  in_1 : Inport
  Constant1 : Constant  Value=inf
  Demux : Demux  Outputs=3
      settings: DisplayOption=none
  Fcn : Fcn  Expr=1/sqrt(u)
  Gain : Gain  Gain=-1  SaturateOnIntegerOverflow=on  OutDataTypeStr=Inherit: Same as input  ParamDataTypeStr=Inherit: Same as input
  Mux : Mux  Inputs=3
  Product{,1..5} (6 alike) : Product  InputSameDT=on  RndMeth=Zero  SaturateOnIntegerOverflow=on  OutDataTypeStr=Inherit: Same as first input
  Sum6 : Sum  Inputs=+++  InputSameDT=on  SaturateOnIntegerOverflow=on  OutDataTypeStr=Inherit: Same as first input
  Switch : Switch
  out_1 : Outport  InitialOutput=0
  wires:
  Sum6/1 -> Gain/1, Switch/3
  Constant1/1 -> Switch/1
  Product5/1 -> Mux/3
  Product3/1 -> Mux/1
  Product4/1 -> Mux/2
  Demux/2 -> Product4/1, Product1/1, Product1/2
  Demux/3 -> Product5/1, Product2/2, Product2/1
  Demux/1 -> Product/2, Product/1, Product3/1
  Product1/1 -> Sum6/2
  Product/1 -> Sum6/1
  Product2/1 -> Sum6/3
  Mux/1 -> out_1/1
  in_1/1 -> Demux/1
  Gain/1 -> Switch/2
  Switch/1 -> Fcn/1
  Fcn/1 -> Product5/2, Product3/2, Product4/2

== system observerModel_MS/Internal Model of Otoliths/Otolith ==
  in_1 : Inport
  Transfer Fcn3 : TransferFcn  Denominator=[1/(2*pi*f_oto) 1]
  out_1 : Outport  InitialOutput=0
  wires:
  in_1/1 -> Transfer Fcn3/1
  Transfer Fcn3/1 -> out_1/1

== system observerModel_MS/Internal Model of Otoliths/Otolith1 ==
  in_1 : Inport
  Transfer Fcn3 : TransferFcn  Denominator=[1/(2*pi*f_oto) 1]
  out_1 : Outport  InitialOutput=0
  wires:
  in_1/1 -> Transfer Fcn3/1
  Transfer Fcn3/1 -> out_1/1

== system observerModel_MS/Internal Model of Otoliths/Otolith2 ==
  in_1 : Inport
  Transfer Fcn3 : TransferFcn  Denominator=[1/(2*pi*f_oto) 1]
  out_1 : Outport  InitialOutput=0
  wires:
  Transfer Fcn3/1 -> out_1/1
  in_1/1 -> Transfer Fcn3/1

== system observerModel_MS/Motion Sickness Dynamics/Oman 1 ==
  note: Ks = 5, Ts = 600sec, ns = 2
  note: Tf = 60sec, nf = 2
  note: if nf = 2, as Oman has it
  In1 : Inport
  Add1 : Sum
  Product : Product
  Transfer Fcn : TransferFcn  Numerator=[Kfast]  Denominator=[beta1^2 2*df*beta1 1]
  Transfer Fcn2 : TransferFcn  Denominator=[beta2^2 2*beta2 1]
  I(t) : Outport  VectorParamsAs1DForOutWhenUnconnected=off
  F(t) : Outport  Port=2  VectorParamsAs1DForOutWhenUnconnected=off
  S(t) : Outport  Port=3  VectorParamsAs1DForOutWhenUnconnected=off
  wires:
  Add1/1 -> I(t)/1  "I(t)"
  Transfer Fcn2/1 -> S(t)/1, Product/2, Add1/2  "S(t)"
  Transfer Fcn/1 -> Add1/1, F(t)/1  "F(t)"
  In1/1 -> Transfer Fcn2/1, Product/1
  Product/1 -> Transfer Fcn/1

== system observerModel_MS/Otoliths/X Graviceptor ==
  in_1 : Inport
  Adaptation : TransferFcn  Numerator=[oto_Ka(1)*oto_a(1) 1]  Denominator=[oto_a(1) 1]
  Low Pass Filter : TransferFcn  Denominator=[1/(2*pi*f_oto) 1]
  New Otolith model : TransferFcn  Numerator=[333 33.3]  Denominator="[0.08  5.016 1]"
  Scope{,1..3} (4 alike) : Scope
  X Graviceptor : TransferFcn  Numerator=[oto_Ka(1)*oto_a(1) 1]  Denominator=[oto_a(1)*1/(2*pi*f_oto) (1/(2*pi*f_oto)+oto_a(1)) 1]
  out_1 : Outport  InitialOutput=0
  wires:
  in_1/1 -> Low Pass Filter/1, X Graviceptor/1, Adaptation/1, New Otolith model/1
  Low Pass Filter/1 -> out_1/1, Scope2/1
  X Graviceptor/1 -> Scope/1
  Adaptation/1 -> Scope1/1
  New Otolith model/1 -> Scope3/1

== system observerModel_MS/Otoliths/Y Graviceptor ==
  in_1 : Inport
  Adaptation : TransferFcn  Numerator=[oto_Ka(2)*oto_a(2) 1]  Denominator=[oto_a(2) 1]
  Low Pass Filter : TransferFcn  Denominator=[1/(2*pi*f_oto) 1]
  New Otolith model : TransferFcn  Numerator=[333 33.3]  Denominator="[0.08  5.016 1]"
  Scope{,1..3} (4 alike) : Scope
  X Graviceptor : TransferFcn  Numerator=[oto_Ka(2)*oto_a(2) 1]  Denominator=[oto_a(2)*1/(2*pi*f_oto) (1/(2*pi*f_oto)+oto_a(2)) 1]
  out_1 : Outport  InitialOutput=0
  wires:
  in_1/1 -> Low Pass Filter/1, X Graviceptor/1, Adaptation/1, New Otolith model/1
  Low Pass Filter/1 -> out_1/1, Scope2/1
  X Graviceptor/1 -> Scope/1
  Adaptation/1 -> Scope1/1
  New Otolith model/1 -> Scope3/1

== system observerModel_MS/Otoliths/Z Graviceptor ==
  in_1 : Inport
  Adaptation : TransferFcn  Numerator=[oto_Ka(3)*oto_a(3) 1]  Denominator=[oto_a(3) 1]
  Low Pass Filter : TransferFcn  Denominator=[1/(2*pi*f_oto) 1]
  New Otolith model : TransferFcn  Numerator=[333 33.3]  Denominator="[0.08  5.016 1]"
  Scope{,1..3} (4 alike) : Scope
  X Graviceptor : TransferFcn  Numerator=[oto_Ka(3)*oto_a(3) 1]  Denominator=[oto_a(3)*1/(2*pi*f_oto) (1/(2*pi*f_oto)+oto_a(3)) 1]
  out_1 : Outport  InitialOutput=0
  wires:
  Low Pass Filter/1 -> out_1/1, Scope2/1
  X Graviceptor/1 -> Scope/1
  Adaptation/1 -> Scope1/1
  New Otolith model/1 -> Scope3/1
  in_1/1 -> Low Pass Filter/1, X Graviceptor/1, Adaptation/1, New Otolith model/1

== system observerModel_MS/Quaternion Rotator/Head to Limbic Angular Velocity Transform ==
  omega_head : Inport
  D_Cos : Inport  Port=2
  Gain : Gain  Gain=-1
  Product1 : Product  Multiplication=Matrix(*)  RndMeth=Zero
  Quaternion Integrator1 : Subsystem
  Quaternion to Direction Cosine1 : Subsystem
  Transform Axes : Subsystem
  Transpose : Math  Operator=transpose  SignedPower=on
  R_limbic : Outport
  wires:
  Quaternion Integrator1/1(q) -> Quaternion to Direction Cosine1/1(q)
  Quaternion to Direction Cosine1/1(D_Cos) -> R_limbic/1
  omega_head/1 -> Product1/2
  Transpose/1 -> Product1/1
  D_Cos/1 -> Transpose/1
  Product1/1 -> Transform Axes/1(limbic_cord)
  Transform Axes/1(VR_cord) -> Gain/1
  Gain/1 -> Quaternion Integrator1/1(omega_limbic)

== system observerModel_MS/Quaternion Rotator/Quaternion Integrator ==
  omega_head : Inport
  Demux1 : Demux
  Gain : Gain  Gain=1/delta_t
  Mux1 : Mux
  delta_q : Subsystem
  q0 : Integrator  InitialCondition=Q0(1)
  q1 : Integrator  InitialCondition=Q0(2)
  q2 : Integrator  InitialCondition=Q0(3)
  q3 : Integrator  InitialCondition=Q0(4)
  q : Outport
  wires:
  Demux1/1 -> q0/1
  q0/1 -> Mux1/1
  Demux1/2 -> q1/1
  q1/1 -> Mux1/2
  Demux1/3 -> q2/1
  q2/1 -> Mux1/3
  Demux1/4 -> q3/1
  q3/1 -> Mux1/4
  Mux1/1 -> delta_q/2(q), q/1
  Gain/1 -> Demux1/1
  delta_q/1(delta_q) -> Gain/1
  omega_head/1 -> delta_q/1(omega)
